simulink model "pulse66"  (R2016a)
settings: Solver=FixedStepAuto  SolverMode=SingleTasking  StartTime=0.0  StopTime=0.2  FixedStep=1e-4  RelTol=1e-3
libraries: powerlib x16, electricdrivelib x1
settings Model: Creator=DELL  LastModifiedBy=Muhammad
settings DebuggingCC: SFUnexpectedBacktrackingDiag=error  SFNoUnconditionalDefaultTransitionDiag=error
settings GRTTargetCC: TargetLangStandard=C99 (ISO)  GeneratePreprocessorConditionals=Use local settings
settings ConfigComp: CovMetricSettings=dwe  CovHtmlReporting=off  CovSaveCumulativeToWorkspaceVar=off  CovSaveSingleToWorkspaceVar=off  CovExternalEMLEnable=on

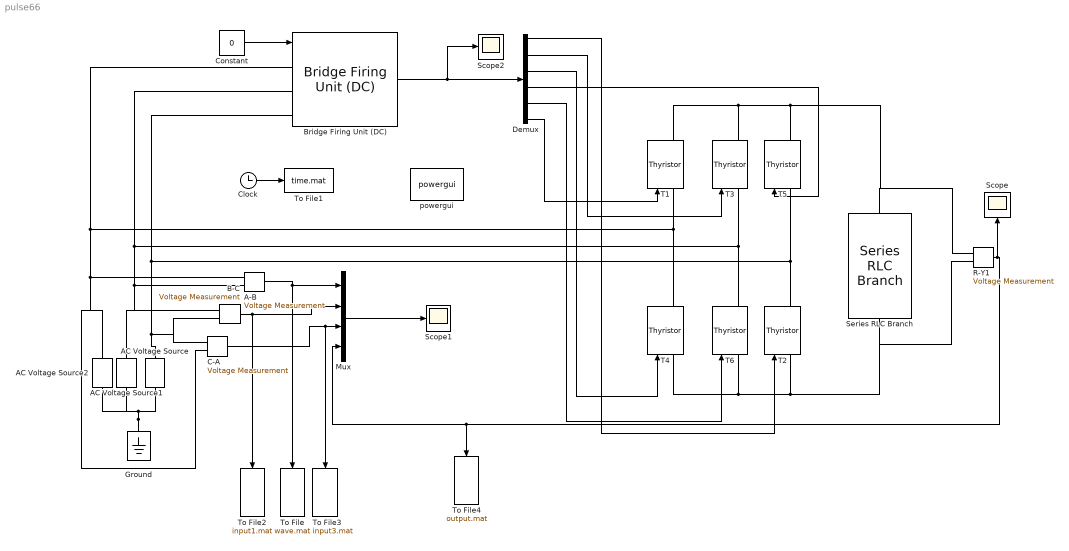
== system pulse66 ==
  A-B : powerlib/Measurements/Voltage Measurement  PhasorSimulation=off  OutputType=Complex  PSBequivalent=0
  AC Voltage Source : powerlib/Electrical Sources/AC Voltage Source  Amplitude=18  Phase=-120  Frequency=60  SampleTime=0  Measurements=None  BusType=swing  Pref=10e3  Qref=0  Qmin=-inf  Qmax=+inf
  AC Voltage Source1 : powerlib/Electrical Sources/AC Voltage Source  Amplitude=18  Phase=120  Frequency=60  SampleTime=0  Measurements=None  BusType=swing  Pref=10e3  Qref=0  Qmin=-inf  Qmax=+inf
  AC Voltage Source2 : powerlib/Electrical Sources/AC Voltage Source  Amplitude=18  Phase=0  Frequency=60  SampleTime=0  Measurements=None  BusType=swing  Pref=10e3  Qref=0  Qmin=-inf  Qmax=+inf
  B-C : powerlib/Measurements/Voltage Measurement  PhasorSimulation=off  OutputType=Complex  PSBequivalent=0
  Bridge Firing Unit (DC) : electricdrivelib/Fundamental Drive Blocks/Bridge Firing Unit (DC)  OverrideUsingVariant=AC_Detailed_two quadrant  detailLevel=Detailed  nbPhases=3  numQuad=2  x4=60  x9=2  Ts=10
  C-A : powerlib/Measurements/Voltage Measurement  PhasorSimulation=off  OutputType=Complex  PSBequivalent=0
  Clock : Clock
  Constant : Constant  Value=0
  Demux : Demux  Outputs=6
  Ground : powerlib/Elements/Ground  LConnTagsString=a
  Mux : Mux
  R-Y1 : powerlib/Measurements/Voltage Measurement  PhasorSimulation=off  OutputType=Complex  PSBequivalent=0
  Scope : Scope
  Scope1 : Scope
  Scope2 : Scope
  Series RLC Branch : powerlib/Elements/Series RLC Branch  LConnTagsString=__new0  RConnTagsString=__new0  BranchType=RL  Resistance=10  Inductance=0  SetiL0=off  InitialCurrent=0  Capacitance=1e-6  Setx0=off  InitialVoltage=0  Measurements=Branch voltage and current
  T{1..6} (6 alike) : powerlib/Power Electronics/Thyristor  Ron=0.001  Lon=0  Vf=0.8  IC=0  Rs=500  Cs=250e-9  Measurements=on
  To File : ToFile  Filename=wave.mat  MatrixName=wave
  To File1 : ToFile  Filename=time.mat  MatrixName=time
  To File2 : ToFile  Filename=input1.mat  MatrixName=input1
  To File3 : ToFile  Filename=input3.mat  MatrixName=input3
  To File4 : ToFile  Filename=output.mat  MatrixName=output
  powergui : powerlib/powergui  Priority=1  SimulationMode=Continuous  SolverType=Tustin/Backward Euler (TBE)  SampleTime=50e-6  frequency=60  SPID=off  DisableSnubberDevices=off  DisableRonSwitches=off  DisableVfSwitches=off  SwTol=0  DisplayEquations=off  Interpol=off  ExternalGateDelay=off  methode=off  Ts=10  FunctionMessages=off  echomessages=off  HookPort=off  EnableUseOfTLC=off  x0status=blocks  frequencyindice=0  Pbase=100e6  ErrMax=1e-4  Iterations=50  UnitsV=kV  UnitsW=MW  buscounter=0  RestoreLinks=warning  ResistiveCurrentMeasurement=off  Frange=[0:2:500]  Ylog=off  Xlog=on  ShowGrid=off  save=off  variable=ZData  structure=0  ZoomFFT=off  StartTime=0.0  cycles=1  DisplayStyle=1  fundamental=60  FreqAxis=off  MaxFrequency=1000  frequencyindicesteady=1  RmsSteady=1  display=off
  wires:
  Demux/1 -> T2/1
  Demux/2 -> T3/1
  Demux/3 -> T4/1
  Demux/4 -> T5/1
  Demux/5 -> T6/1
  Demux/6 -> T1/1
  Mux/1 -> Scope1/1
  A-B/1 -> Mux/1, To File/1
  B-C/1 -> Mux/2, To File2/1
  C-A/1 -> Mux/3, To File3/1
  Constant/1 -> Bridge Firing Unit (DC)/1
  Bridge Firing Unit (DC)/1 -> Scope2/1, Demux/1
  Clock/1 -> To File1/1
  R-Y1/1 -> To File4/1, Mux/4, Scope/1
  connections:
  T1/LConn1 -- Bridge Firing Unit (DC)/LConn1 -- AC Voltage Source2/RConn1 -- C-A/LConn2 -- A-B/LConn1 -- T4/RConn1
  T3/LConn1 -- Bridge Firing Unit (DC)/LConn2 -- AC Voltage Source1/RConn1 -- B-C/LConn1 -- A-B/LConn2 -- T6/RConn1
  T4/LConn1 -- T6/LConn1 -- Series RLC Branch/RConn1 -- R-Y1/LConn2 -- T2/LConn1
  T1/RConn1 -- T3/RConn1 -- Series RLC Branch/LConn1 -- R-Y1/LConn1 -- T5/RConn1
  Ground/LConn1 -- AC Voltage Source2/LConn1 -- AC Voltage Source1/LConn1 -- AC Voltage Source/LConn1
  T5/LConn1 -- C-A/LConn1 -- B-C/LConn2 -- AC Voltage Source/RConn1 -- Bridge Firing Unit (DC)/LConn3 -- T2/RConn1
